simulink model "Body_model"  (R2025b)
settings: Solver=VariableStepAuto  StartTime=0.0  StopTime=3600*9  RelTol=1e-3
InitFcn:
  | run('Body_varibles.m')
values from neighbouring files (symbols this model uses):
  A_BSA = 1.89    [Body_varibles.m]
  A_eff = (0.10 * A_BSA) + (0.15 * A_BSA * 0.50)    (= 0.33075)    [Body_varibles.m]
  ambient_temp = 21    [Body_varibles.m]
  C_core = 20 * 3470    (= 69400)    [Body_varibles.m]
  C_periph = 35 * 2500    (= 87500)    [Body_varibles.m]
  intial_start_of_GA = 3600/2    (= 1800)    [Body_varibles.m]
  k_blood_dilated = 50    [Body_varibles.m]
  Q_loss_base = 23    [Body_varibles.m]
  Q_met_awake = 101    [Body_varibles.m]
  Q_met_GA = Q_met_awake * (1 - 0.25)    (= 75.75)    [Body_varibles.m]
  T_core_0 = Core_temp    (= 37)    [Body_varibles.m]
  T_periph_0 = peripheral_temp    (= 34)    [Body_varibles.m]
undefined symbols (not defined in the file or in its folder): c_air, f_resp, rho_air, T_core_target, V_tidal
libraries: simulink x1
settings Model: Creator=Jack Hamer  LastModifiedBy=Jack Hamer
settings DebuggingCC: AlgebraicLoopMsg=none

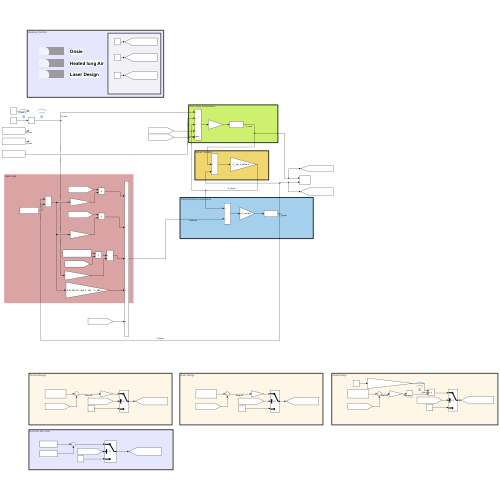
[thumbnail: Simulink's stored preview of the top-level diagram]
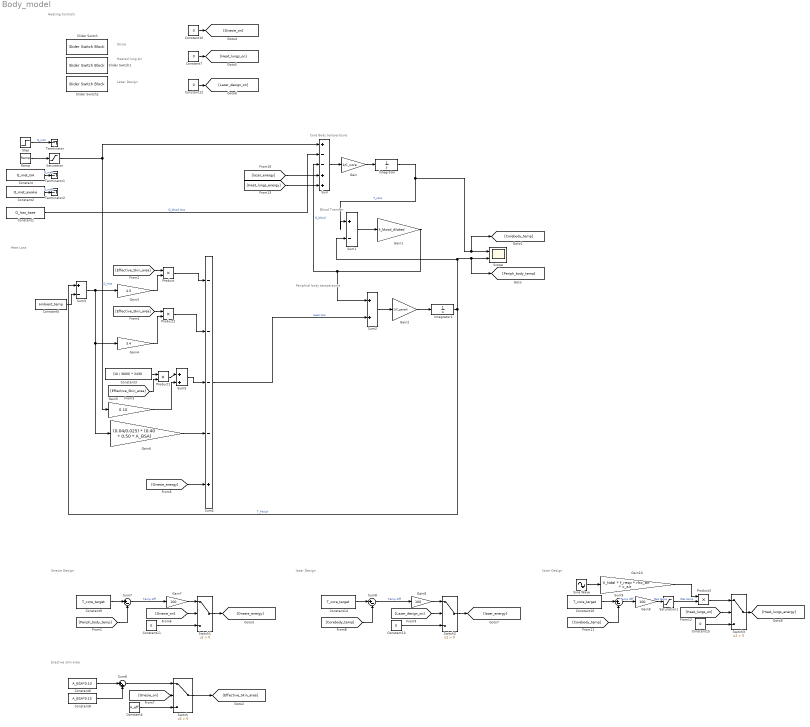
== system Body_model ==
  note: Onesie Design
  note: Onsie
  note: Heating Controls
  note: Blood Transfer
  note: Periphral body temperature
  note: Core Body temperature
  note: Heat Loss
  note: Heated lung Air
  note: Laser Design
  note: Evective skin area
  note: lazer Design
  note: lazer Design
  Constant : Constant  Value=Q_met_GA
  Constant1 : Constant  Value=Q_loss_base
  Constant{7,10..13,15} (6 alike) : Constant  Value=0
  Constant14 : Constant  Value=T_core_target
  Constant16 : Constant  Value=T_core_target
  Constant2 : Constant  Value=Q_met_awake
  Constant3 : Constant  Value=(10 / 3600) * 2430
  Constant4 : Constant  Value=A_eff
  Constant5 : Constant  Value=ambient_temp
  Constant6 : Constant  Value=A_BSA*0.10
  Constant8 : Constant  Value=A_BSA*0.15
  Constant9 : Constant  Value=T_core_target
  Gain : Gain  Gain=1/C_core
  Gain1 : Gain  Gain=k_blood_dilated
  Gain10 : Gain  Gain=V_tidal * f_resp * rho_air * c_air
  Gain2 : Gain  Gain=1/C_periph
  Gain3 : Gain  Gain=4.5
  Gain4 : Gain  Gain=3.4
  Gain5 : Gain  Gain=0.10
  Gain6 : Gain  Gain=(0.04/0.025) * (0.40 * 0.50 * A_BSA)
  Gain7 : Gain  Gain=100
  Gain8 : Gain  Gain=100
  Gain9 : Gain  Gain=100
  Integrator : Integrator  InitialCondition=T_core_0  LimitOutput=on
  Integrator1 : Integrator  InitialCondition=T_periph_0  LimitOutput=on
  Product{,1..3} (4 alike) : Product
  Ramp : simulink/Sources/Ramp  slope=(-Q_met_awake+Q_met_GA)/60  start=intial_start_of_GA  InitialOutput=101
  Saturation : Saturate  UpperLimit=Q_met_awake  LowerLimit=Q_met_GA
  Saturation1 : Saturate  UpperLimit=100  LowerLimit=ambient_temp
  Scope : Scope  NumInputPorts=2
      settings: ActiveDisplayYMinimum=32.34694592426883  ActiveDisplayYMaximum=38.455300774684233
  Sine Wave : Sin  Frequency=2*pi*f_resp  SampleTime=0
  Slider Switch : SliderSwitchBlock
  Slider Switch1 : SliderSwitchBlock
  Slider Switch2 : SliderSwitchBlock
  Step : Step  Time=intial_start_of_GA  Before=Q_met_awake  After=Q_met_GA  SampleTime=0
  Sum : Sum  Inputs=+--++
  Sum{1,7..9} (4 alike) : Sum  Inputs=|+-
  Sum2 : Sum
  Sum3 : Sum  Inputs=+-
  Sum4 : Sum  Inputs=----+
  Sum5 : Sum  Inputs=|++
  Sum6 : Sum  Inputs=|++
  Switch{,1..3} (4 alike) : Switch  Criteria=u2 > Threshold  SaturateOnIntegerOverflow=off  InputSameDT=off
  Terminator : Terminator
  Terminator1 : Terminator
  Terminator2 : Terminator
  wires:
  Saturation/1 -> Gain5/1, Sum/1  "Q_met"
  Constant1/1 -> Sum/2  "Q_blood loss"
  Sum/1 -> Gain/1
  Gain/1 -> Integrator/1
  Integrator/1 -> Sum1/1, [Corebody_temp], Scope/1  "T_core"
  Sum1/1 -> Gain1/1
  Gain1/1 -> Sum2/1, Sum/3  "Q_blood"
  Sum4/1 -> Sum2/2  "Heat loss"
  Sum2/1 -> Gain2/1
  Gain2/1 -> Integrator1/1
  Integrator1/1 -> [Periph_body_temp], Scope/2, Sum1/2, Sum3/1  "T_Periph"
  Constant5/1 -> Sum3/2
  Sum3/1 -> Gain4/1, Gain6/1, Gain3/1
  Product/1 -> Sum4/1
  Product2/1 -> Sum4/2
  Sum5/1 -> Sum4/3
  Gain6/1 -> Sum4/4
  Constant3/1 -> Product1/1
  Gain5/1 -> Sum5/2
  Ramp/1 -> Saturation/1
  Step/1 -> Terminator/1  "Q_met"
  Constant/1 -> Terminator1/1  "Q_met"
  Constant2/1 -> Terminator2/1  "Q_met"
  Gain3/1 -> Product/2
  [Effective_Skin_area] -> Product/1
  Constant4/1 -> Switch/3
  [Effective_Skin_area] -> Product1/2
  Product1/1 -> Sum5/1
  [Effective_Skin_area] -> Product2/1
  Gain4/1 -> Product2/2
  Constant6/1 -> Sum6/1
  Switch/1 -> [Effective_Skin_area]
  [Onesie_on] -> Switch/2
  Sum6/1 -> Switch/1
  Constant8/1 -> Sum6/2
  Gain7/1 -> Switch1/1
  Sum7/1 -> Gain7/1  "Temp diff"
  [Onesie_energy] -> Sum4/5
  Constant9/1 -> Sum7/1
  [Periph_body_temp] -> Sum7/2
  Constant11/1 -> Switch1/3
  Switch1/1 -> [Onesie_energy]
  Constant10/1 -> [Onesie_on]
  [Onesie_on] -> Switch1/2
  Constant7/1 -> [Heat_lungs_on]
  Constant12/1 -> [Lazer_design_on]
  [Lazer_design_on] -> Switch2/2
  Switch2/1 -> [lazer_energy]
  Constant13/1 -> Switch2/3
  [Corebody_temp] -> Sum8/2
  Constant14/1 -> Sum8/1
  Sum8/1 -> Gain8/1  "Temp diff"
  Gain8/1 -> Switch2/1
  [lazer_energy] -> Sum/4
  Saturation1/1 -> Product3/2  "Gas temp"
  Sum9/1 -> Gain9/1  "Temp diff"
  Constant16/1 -> Sum9/1
  [Corebody_temp] -> Sum9/2
  Constant15/1 -> Switch3/3
  Switch3/1 -> [Heat_lungs_energy]
  [Heat_lungs_on] -> Switch3/2
  Sine Wave/1 -> Gain10/1
  Product3/1 -> Switch3/1
  Gain10/1 -> Product3/1
  [Heat_lungs_energy] -> Sum/5
  Gain9/1 -> Saturation1/1  "Gas temp"
